simulink model "untitled"  (R2023a)
settings: Solver=VariableStepAuto  StartTime=0.0  StopTime=10.0  RelTol=1e-3
values from neighbouring files (symbols this model uses):
  H = 100    [Calculos00_OriginalIgnacio.m]    (also in Calculos02_Vnoladetrim.m; Calculos03_TablaTrimados.m; GenerateDataset_v0.m = vH(j); PI_0_OnlyOneController_V20.m = vH(j))
  V = 12    [Calculos00_OriginalIgnacio.m]    (also in Calculos02_Vnoladetrim.m = 6; Calculos03_TablaTrimados.m = vV(k); GenerateDataset_v0.m = vV(i); PI_0_OnlyOneController_V20.m = vV(i))
libraries: simulink x1
settings Model: Creator=ignac  LastModifiedBy=ignac

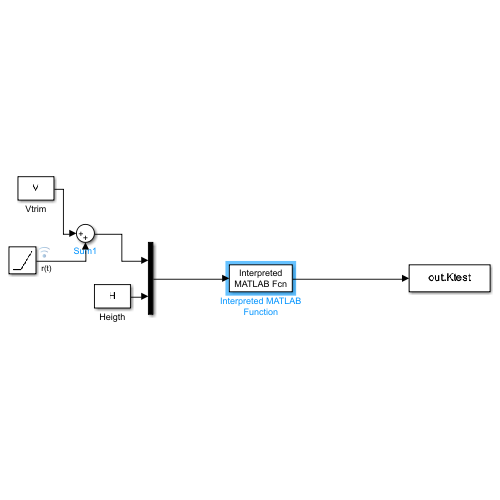
[thumbnail: Simulink's stored preview of the top-level diagram]
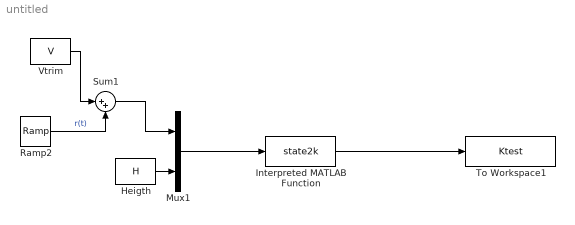
== system untitled ==
  Heigth : Constant  Value=H
  Interpreted MATLAB Function : MATLABFcn  MATLABFcn=state2k  OutputDimensions=[2,5]  Output1D=off
  Mux1 : Mux  Inputs=2
  Ramp2 : simulink/Sources/Ramp  slope=1  start=0  InitialOutput=0
  Sum1 : Sum  Inputs=|++
  To Workspace1 : ToWorkspace  VariableName=Ktest  SaveFormat=Timeseries  SampleTime=-1
      settings: Save2DSignal=2-D array (concatenate along first dimension)
  Vtrim : Constant  Value=V
  wires:
  Heigth/1 -> Mux1/2
  Sum1/1 -> Mux1/1
  Mux1/1 -> Interpreted MATLAB Function/1
  Ramp2/1 -> Sum1/2  "r(t)"
  Vtrim/1 -> Sum1/1
  Interpreted MATLAB Function/1 -> To Workspace1/1
